simulink library "carnot"  (R2018b)
settings: Solver=VariableStepAuto  StartTime=0.0  StopTime=10.0  RelTol=1e-3
undefined symbols (not defined in the file or in its folder): A, A_earth, acol, Acol, ActPower1, ActPower2, ActPower3, Ad, Ad0, Ar, Au, Au0, Azimuth_Angle, B, Bd, Bd0, Br, Bu, Bu0, C, c1, c2, c3, c33, c4, c5, c6, CarnotCallbacks_Density, CarnotCallbacks_Enthalpy, CarnotCallbacks_Enthalpy2Temperature, CarnotCallbacks_Entropy, CarnotCallbacks_Evaporation_Enthalpy, CarnotCallbacks_GlobalMessageLevel, CarnotCallbacks_Grashof, CarnotCallbacks_Heat_Capacity, CarnotCallbacks_Kinematic_Viscosity, CarnotCallbacks_PMV_PPD, CarnotCallbacks_Prandtl, CarnotCallbacks_Saturation_Property, CarnotCallbacks_Saturation_Temperature, CarnotCallbacks_Saturation_Value_Water, CarnotCallbacks_Specific_Volume, CarnotCallbacks_Thermal_Conductivity, CarnotCallbacks_Vapour_Content, CarnotCallbacks_Vapour_Pressure, Cd, Cdl, Cr, Cu, Davies, Dd, DE_TRY2010_04_averageYear, delta_grd, density, DiameterLastPiece, dl, DPConstant, DPLinear, DPQuadratic, Dr ... (+59)
libraries: $bdroot x429, simulink x36, simulink_extras x12
(part 4 of 22)

== system carnot/Basic/Electric ==
  EBCreator : Subsystem  InitFcn=load('EB.mat');  mask(EBCreator){Inport_ID=on, Inport_f=on, Inport_v1=on, Inport_p1=on, Inport_pf1=on, Inport_v2=on, Inport_p2=on, Inport_pf2=on, Inport_v3=on, Inport_p3=on, Inport_pf3=on, ID=4, f=50, v1=230, p1=0, pf1=1, v2=230, p2=0, pf2=1, v3=230, p3=0, pf3=1, Annotation_ID=off, Annotation_f=off, Annotation_v1=off, Annotation_p1=off, Annotation_pf1=off, Annotation_v2=off, Annotation_p2=off, Annotation_pf2=off, Annotation_v3=off, Annotation_p3=off, Annotation_pf3=on}
      mask prompts: Inport_ID "ID as inport"; Inport_f "frequency as inport"; Inport_v1 "voltage line 1 as inport"; Inport_p1 "active power line 1 as inport"; Inport_pf1 "power factor line 1 as inport"; Inport_v2 "voltage line 2 as inport"; Inport_p2 "active power line 1 as inport"; Inport_pf2 "power factor line 2 as inport"; Inport_v3 "voltage line 3 as inport"; Inport_p3 "active power line 3 as inport"; Inport_pf3 "power factor line 3 as inport"; ID "ID [1]"; f "frequency [Hz]"; v1 "voltage line 1 [V]"; p1 "active power line 1 [W]"; pf1 "power factor line 1 [1]"; v2 "voltage line 2 [V]"; p2 "active power line 2 [W]"; pf2 "power factor line 2 [1]"; v3 "voltage line 3 [V]"; p3 "active power line 3 [W]"; pf3 "power factor line 3 [1]"; Annotation_ID "ID as annotation"; Annotation_f "Frequency as annotation"; Annotation_v1 "voltage line 1 as annotation"; Annotation_p1 "active power line 1 as annotation"; Annotation_pf1 "fluid type as annotation"; Annotation_v2 "voltage line 2 as annotation"; Annotation_p2 "active power line 2 as annotation"; Annotation_pf2 "power factor line 2 as annotation"; Annotation_v3 "voltage line 3 as annotation"; Annotation_p3 "voltage line 3 as annotation"; Annotation_pf3 "power factor line 3 as annotation"
      mask help:
      | This block creates an EB from input signals.
      | ID is:
      | 1  Power only
      | 2  DC
      | 3  AC_1Phase
      | 4  AC_3Phase
      mask init:
      | CarnotCallbacks_EBCreator('CreateInports', gcb);
      mask Help: web(fullfile(path_carnot('help'),'EBCreator.html'),'-helpbrowser')
      mask Callback Inport_ID:
      | CarnotCallbacks_EBCreator('CreateMaskVisibilities', gcb);
      | CarnotCallbacks_EBCreator('CreateMaskAnnotations', gcb);
      mask Callback Inport_f:
      | CarnotCallbacks_EBCreator('CreateMaskVisibilities', gcb);
      | CarnotCallbacks_EBCreator('CreateMaskAnnotations', gcb);
      mask Callback Inport_v1:
      | CarnotCallbacks_EBCreator('CreateMaskVisibilities', gcb);
      | CarnotCallbacks_EBCreator('CreateMaskAnnotations', gcb);
      mask Callback Inport_p1:
      | CarnotCallbacks_EBCreator('CreateMaskVisibilities', gcb);
      | CarnotCallbacks_EBCreator('CreateMaskAnnotations', gcb);
      mask Callback Inport_pf1:
      | CarnotCallbacks_EBCreator('CreateMaskVisibilities', gcb);
      | CarnotCallbacks_EBCreator('CreateMaskAnnotations', gcb);
      mask Callback Inport_v2:
      | CarnotCallbacks_EBCreator('CreateMaskVisibilities', gcb);
      | CarnotCallbacks_EBCreator('CreateMaskAnnotations', gcb);
      mask Callback Inport_p2:
      | CarnotCallbacks_EBCreator('CreateMaskVisibilities', gcb);
      | CarnotCallbacks_EBCreator('CreateMaskAnnotations', gcb);
      mask Callback Inport_pf2:
      | CarnotCallbacks_EBCreator('CreateMaskVisibilities', gcb);
      | CarnotCallbacks_EBCreator('CreateMaskAnnotations', gcb);
      mask Callback Inport_v3:
      | CarnotCallbacks_EBCreator('CreateMaskVisibilities', gcb);
      | CarnotCallbacks_EBCreator('CreateMaskAnnotations', gcb);
      mask Callback Inport_p3:
      | CarnotCallbacks_EBCreator('CreateMaskVisibilities', gcb);
      | CarnotCallbacks_EBCreator('CreateMaskAnnotations', gcb);
      mask Callback Inport_pf3:
      | CarnotCallbacks_EBCreator('CreateMaskVisibilities', gcb);
      | CarnotCallbacks_EBCreator('CreateMaskAnnotations', gcb);
      mask Callback ID: CarnotCallbacks_EBCreator('CreateMaskAnnotations', gcb);
      mask Callback f: CarnotCallbacks_EBCreator('CreateMaskAnnotations', gcb);
      mask Callback v1: CarnotCallbacks_EBCreator('CreateMaskAnnotations', gcb);
      mask Callback p1: CarnotCallbacks_EBCreator('CreateMaskAnnotations', gcb);
      mask Callback pf1: CarnotCallbacks_EBCreator('CreateMaskAnnotations', gcb);
      mask Callback v2: CarnotCallbacks_EBCreator('CreateMaskAnnotations', gcb);
      mask Callback p2: CarnotCallbacks_EBCreator('CreateMaskAnnotations', gcb);
      mask Callback pf2: CarnotCallbacks_EBCreator('CreateMaskAnnotations', gcb);
      mask Callback v3: CarnotCallbacks_EBCreator('CreateMaskAnnotations', gcb);
      mask Callback p3: CarnotCallbacks_EBCreator('CreateMaskAnnotations', gcb);
      mask Callback pf3: CarnotCallbacks_EBCreator('CreateMaskAnnotations', gcb);
      mask Callback Annotation_ID: CarnotCallbacks_EBCreator('CreateMaskAnnotations', gcb);
      mask Callback Annotation_f: CarnotCallbacks_EBCreator('CreateMaskAnnotations', gcb);
      mask Callback Annotation_v1: CarnotCallbacks_EBCreator('CreateMaskAnnotations', gcb);
      mask Callback Annotation_p1: CarnotCallbacks_EBCreator('CreateMaskAnnotations', gcb);
      mask Callback Annotation_pf1: CarnotCallbacks_EBCreator('CreateMaskAnnotations', gcb);
      mask Callback Annotation_v2: CarnotCallbacks_EBCreator('CreateMaskAnnotations', gcb);
      mask Callback Annotation_p2: CarnotCallbacks_EBCreator('CreateMaskAnnotations', gcb);
      mask Callback Annotation_pf2: CarnotCallbacks_EBCreator('CreateMaskAnnotations', gcb);
      mask Callback Annotation_v3: CarnotCallbacks_EBCreator('CreateMaskAnnotations', gcb);
      mask Callback Annotation_p3: CarnotCallbacks_EBCreator('CreateMaskAnnotations', gcb);
      mask Callback Annotation_pf3: CarnotCallbacks_EBCreator('CreateMaskAnnotations', gcb);
      mask DialogControl ParameterTabVar0 Prompt: Settings
      mask DialogControl ParameterTabVar01 Prompt: Values
      mask DialogControl ParameterTabVar012 Prompt: Annotations
  basic_EB : Subsystem  InitFcn=load('EB.mat')  mask(basic_EB){eID=Power only, f=50, v1=230, p1=0, pf1=1, v2=230, p2=0, pf2=1, v3=230, p3=0, pf3=1}
      mask prompts: eID "ID for electric calculation"; f "frequency [Hz]"; v1 "voltage to ground [V]"; p1 "active  power [VA]"; pf1 "power factor[-]"; v2 "voltage to ground [V]"; p2 "active  power [VA]"; pf2 "power factor[-]"; v3 "voltage to ground [V]"; p3 "active  power [VA]"; pf3 "power factor[-]"
      mask help: Create a constant Electric Bus.
      mask Help: web(fullfile(path_carnot('help'),'basic_EB.html'),'-helpbrowser')
      mask TypeOptions eID: ID/eID
      mask TypeOptions f: f/Value
      mask TypeOptions v1: v1/Value
      mask TypeOptions p1: p1/Value
      mask TypeOptions pf1: pf1/Value
      mask TypeOptions v2: v2/Value
      mask TypeOptions p2: p2/Value
      mask TypeOptions pf2: pf2/Value
      mask TypeOptions v3: v3/Value
      mask TypeOptions p3: p3/Value
      mask TypeOptions pf3: pf3/Value
      mask DialogControl ParameterTabVar03 Prompt: Common
      mask DialogControl ParameterTabVar0 Prompt: Line 1
      mask DialogControl ParameterTabVar01 Prompt: Line2
      mask DialogControl ParameterTabVar02 Prompt: Line3
  basic_create_EB : Subsystem  InitFcn=load('EB.mat')  mask(basic_create_EB){eID=Power only, f=50, pf1=1, pf2=1, pf3=1}
      mask prompts: eID "ID for electric calculation"; f "frequency [Hz]"; pf1 "power factor line 1 [-]"; pf2 "power factor line 2 [-]"; pf3 "power factor line 3 [-]"
      mask help: Block to create an EB with the variable inputs ActPower and Voltage. The other values can be set as constants in the mask.
      mask Help: web(fullfile(path_carnot('help'),'basic_create_EB.html'),'-helpbrowser')
      mask TypeOptions eID: basic_EB/eID
      mask TypeOptions f: basic_EB/f
      mask TypeOptions pf1: basic_EB/pf1
      mask TypeOptions pf2: basic_EB/pf2
      mask TypeOptions pf3: basic_EB/pf3

== system carnot/Basic/Heat_Transfer ==
  HeatTransfer2Ground_ISO13370 : Subsystem  mask(Heat Transfer to Ground ISO 13370){slabwidth=10, slablength=7, gammat=0, Tmeaninside=23.8, deltathetai=3.8, Tmeanoutside=11, deltathetae=9.3, tshift=319*3600, dwall=0.4, cond_ground=2.0, cp_ground=800, rho_ground=2500, utot=0.183}
      mask prompts: slabwidth "Width of slab in m"; slablength "Length of slab in m"; gammat "Linear thermal transmittance associated with wall/floor junctions [W/mK]"; Tmeaninside "Mean annual inside temperature [°C]"; deltathetai "Annual amplitude of inside temperature [°C]"; Tmeanoutside "Mean annual outside temperature [°C]"; deltathetae "Annual amplitude of outside temperature [°C]"; tshift "Time shift where outside temperature sine-curve shows a mimimum [s]"; dwall "Average thickness of walls inlcuding all layers [m]"; cond_ground "Conductivity of ground [W/(m*K)]"; cp_ground "Capacity of ground [J/(kg*K)]"; rho_ground "Density of ground [kg/m^3]"; utot "Total heat transfer of slab to ground [W/m²/K]"
      mask help:
      | Ground heat transfer for a floor "SLAB ON GROUND" according to ISO 13370:2007.
      | Use function fitSineToTamb to find the weather parameters.
      mask Help: web(fullfile(path_carnot('help'),'Heattransfer2GroundISO.html'),'-helpbrowser')
      mask Display: disp('U(ground)\nISO13370')
  HeatTransfer2Ground_Simple : Subsystem  mask(Heat Transfer to Ground simple Model){Tground=10, UAground=0.2*70}
      mask prompts: Tground "Ground temperature in °C"; UAground "Heat transfer to ground in W/K"
      mask help:
      | Very simple model for the heat transfer of a house to the ground.
      | See Help for details.
      mask Help: web(fullfile(path_carnot('help'),'Heattransfer2Ground_Simple.html'),'-helpbrowser')
  alfa_ceiling : Subsystem  mask(ALFA){active=0, emission_c=0.65, wallsurface=1}
      mask prompts: active "active layer (0 / 1)"; emission_c "Longwave emissivity of surface (0..1)"; wallsurface "Ceiling surface in m²"
      mask help:
      | Convective and radiative heat transfer at the SURFACE OF A HORIZONTAL CEELING.
      | [AIV] : conditions of zone node,
      | Ts : temperature of outdoor wall surface, °C,
      | qdots : specific heat flow into wall construction, W/m^2,
      | [S] : heat and air flow to zone node.
      mask Help: web(fullfile(path_carnot('help'),'alfa_ceiling.html'),'-helpbrowser')
  alfa_floor : Subsystem  mask(ALFA){active=0, emission_f=0.65, wallsurface=1}
      mask prompts: active "active layer (0 / 1)"; emission_f "Longwave emissivity of surface (0..1)"; wallsurface "Floor surface in m²"
      mask help:
      | Convective and radiative heat transfer at the SURFACE OF A HORIZONTAL FLOOR.
      |
      | [AIV] : conditions of zone node,
      | Ts : temperature of wall surface, °C,
      | qdots : specific heat flow into wall construction, W/m^2,
      | [S] : heat and air flow to zone node.
      mask Help: web(fullfile(path_carnot('help'),'alfa_floor.html'),'-helpbrowser')
  alfa_wall_in : Subsystem  mask(ALFA){active=0, emission_in=0.7, wallsurface=1}
      mask prompts: active "Active layer (0 / 1)"; emission_in "Longwave emissivity of surface (0..1)"; wallsurface "Wall surface in m²"
      mask help:
      | Convective and radiative heat transfer at the INDOOR SURFACE of a VERTICAL OUTER WALL.
      |
      | [AIV] : conditions of zone node,
      | Ts : temperature of wall surface, °C,
      | qdots : specific heat flow into wall construction, W/m^2,
      | [S] : heat and air flow to zone node.
      mask Help: web(fullfile(path_carnot('help'),'alfa_wall_in.html'),'-helpbrowser')
  alfa_wall_out : Subsystem  mask(ALFA){pos=0, absorption_out=0.4, emission_out=0.7, wallsurface=1}
      mask prompts: pos "Azimut (south = 0, east = -90) in degrees"; absorption_out "Solar absorption outside (0..1)"; emission_out "Longwave emissivity of surface (0..1)"; wallsurface "Wall surface in m²"
      mask help:
      | Convective and radiative HEAT TRANSFER at the WEATHER EXPOSED SURFACE of an OUTER WALL.
      |
      | [W*] : modified weather data, adapted to height over ground,
      | Ts : temperature of outdoor wall surface, °C,
      | qdots : specific heat flow into wall / window construction, W/m^2.
      mask init:
      | if length(pos) == 1
      |     pos = [90  pos 0]; % pos is [inclination azimut rotation]
      | end
      mask Help: web(fullfile(path_carnot('help'),'alfa_wall_out.html'),'-helpbrowser')
  alfa_window_in : Subsystem  mask(ALFA){type_glazing=double glazing normal, gvalue=0.7, tauzero=0.8, emission_in=1, wallsurface=1, frame=0.1, numlayer=2, shad_type=No shading, tau_shad=0.01, bli_a=0.05, bli_b=1, bli_c=0.05, bli_d=0.05, bli_alpha=90, bli_refl=0.2}
      mask prompts: type_glazing "glazing type"; gvalue "Energy transmission by sunlight (g-value) 0..1"; tauzero "transmittance in visible range of the sunlight [0..1]"; emission_in "Longwave emissivity (0..1)"; wallsurface "Surface of the window (with frame) in m²"; frame "Share of the frame on the surface (0...1)"; numlayer "Number of glass panes"; shad_type "shading type [no Shading/exterior/interior]"; tau_shad "solar transmittance of shading element [0..1]"; bli_a "a  Depth of blind blades [m]"; bli_b "b heigth of blind blades [m]"; bli_c "c distance of "b" to back end of blind blade [m]"; bli_d "d offset between blind blades [m]"; bli_refl "optical reflectance of blind surface [0..1]"
      mask help:
      | Convective and radiative heat transfer at the INDOOR SURFACE OF A VERTICAL WINDOW with 1-4 layers (each 3 ... 8 mm thick).
      |
      | Ts  : temperature of window surface, °C,
      | [sun_t]  : sun data (incidence angle, direct and diffuse radiation
      |     at tilted window surface),
      | [AIV]  : conditions of zone node,
      | qdots  : specific heat flow into window construction, W/m^2,
      | qdot_abs : specific irradiation absorption within window
      |     construction,  W/m^2,
      | [S]  : heat and air flow to zone node.
      mask Help: web(fullfile(path_carnot('help'),'alfa_window_in.html'),'-helpbrowser')
      mask TypeOptions type_glazing: double glazing normal | double glazing  thermal insulation | double glazing combi 73/41 | double glazing combi 50/24 | triple glazing normal | triple glazing  thermal insulation
      mask TypeOptions tauzero: Subsystem/tau(0)/Gain
      mask TypeOptions shad_type: No shading | Exterior Screen | Interior Screen | Venetian Blind
  alfa_window_out : Subsystem  mask(ALFA){pos=0, absorption_out=0.01, emission_out=0.87, frame=0.1}
      mask prompts: pos "Azimut of the surface (South = 0; East = -90)"; absorption_out "Solar absorption of the glass (0...1)"; emission_out "Longwave emissivity (0...1)"; frame "Share of the frame on the surface (0..1)"
      mask help:
      | Convective and radiative heat transfer at the OUTDOOR SURFACE OF A VERTICAL WINDOW.
      | Azimut can be a scalar or a vector with [inclination azimut rotation].
      | [WDB] weather data bus, adapted to height over ground,
      | Ts : temperature of outdoor window surface, °C,
      | g : energetic solar radiation transmittance
      | qdots : specific heat flow into window construction, W/m^2,
      | [sun_t] : sun data (incidence angle, direct and diffuse radiation at tilted window surface).
      mask init:
      | if length(pos) == 1
      |     pos = [90  pos 0]; % pos is [inclination azimut rotation]
      | end
      mask Help: web(fullfile(path_carnot('help'),'alfa_window_out.html'),'-helpbrowser')
  wall_out_IR_radiation : Subsystem

== system carnot/Basic/Hydraulics ==
  ElectricConsumptionPump : Subsystem  mask(Electric Consumption of a Pump){e0=10, e1=10, e2=-1}
      mask prompts: e0 "e0: constant coefficient in W"; e1 "e1: linear coefficient in W*s/kg"; e2 "e2: quadratic coefficient in W*(s/kg)²"
      mask help:
      | The electric consumption of the pump is given by the quadratic equation
      |   Pel = e0 + e1*mdot + e2*mdot^2
      | with
      |   mdot : massflow in kg/s
      |   Pel : electric consumption in W
      mask TypeOptions e0: Constant/Value
      mask TypeOptions e1: Linear/Gain
      mask TypeOptions e2: Quadratic/Gain
      mask Display: disp('Pel = e0\n+ e1*mdot\n+ e2*mdot² ')
  Flow_Mixer_basic : Subsystem  mask(Flow Mixer Basic){}
      mask help:
      | The flow mixer calculated the temperature and massflow of 2 entering flows.
      | The temperature is calculated in the block Mix_T_Mdot.
      | The flow diversion fdiv (feed back to the flow diverter) takes care that the pressure drop in the 2 branches is the same. The resulting pressure drop coefficients are calulated in the s-function mix_flow (uses solve_quadratic_equation in Carlib).
      mask Help: web(fullfile(path_carnot('help'),'Flow_Mixer_basic.html'),'-helpbrowser')
      mask Display: disp('Flow\nMixer')
  Grashof : Subsystem  LoadFcn=CarnotCallbacks_Grashof('LoadFcn');  VariantControl=CarlibClassic  mask(Grashof){DEBUGLEVEL=WARNINGLEVEL, MAXTOTALMESSAGES=inf, MAXCONSECUTIVEMESSAGES=inf, WRITETOFILE=0, FILENAME='errors.txt'}
      mask prompts: DEBUGLEVEL "Debug level"; MAXTOTALMESSAGES "maximum number of total warning"; MAXCONSECUTIVEMESSAGES "maximum number of consecutive warnings"; WRITETOFILE "write messages to file"; FILENAME "filename for error messages"
      mask help:
      | Calculates the Gashof number. You may use the block "GlobalMessageLevel" in the Toolbox to handle the debugging messages.
      | Inputs are:
      | 1   wall temperature - scalar or vector
      | 2   temperature at infinite distance - scalar
      | 3   pressure - scalar
      | 4   fluid type (see below) - scalar
      | 5   fluid_mix - scalar
      | 6   characteristic dimension - scalar
      |
      | FluidType        Remarks
      | 1: water          fluid mix is vapourcontent in the 2-phase region
      | 2: air              fluid mix is (kg water) / (kg dry air)
      | 3: cotton oil       -
      | 4: silicone oil     -
      | 5: water-glycol   fluid mix is volume partition [0..1] of propylen glycol
      | 6: Tyfocor LS     function only available in liquid phase
      | 7: Water Constant = water at 20°C
      | 8: Air Constant = air at 20°C
      mask init:
      | %global debug level
      | [DEBUGLEVEL, MAXTOTALMESSAGES, MAXCONSECUTIVEMESSAGES, WRITETOFILE, FILENAME] = CarnotCallbacks_Grashof('CheckDebugLevels', DEBUGLEVEL, MAXTOTALMESSAGES, MAXCONSECUTIVEMESSAGES, WRITETOFILE, FILENAME);
      mask Help: web(fullfile(path_carnot('help'),'Grashof_mdl.html'),'-helpbrowser')
      mask TypeOptions DEBUGLEVEL: DEBUGLEVEL | INFOLEVEL | WARNINGLEVEL | ERRORLEVEL | FATALLEVEL | NOLEVEL
      mask DialogControl ParameterTabVar0 Prompt: Debugging
  Mix_T_Mdot : Subsystem  InitFcn=load('THB.mat');  mask(mix_temperature){mixcalc=Tmix = (mdot1*T1 + mdot2*T2)/(mdot1+mdot2)}
      mask prompts: mixcalc "Calculation of mixture :"
      mask help:
      | Calculate the temperature of the mixture of two flows. Uses enthalpy balance for humid air. Liquids may be mixed by the (faster and approximate) equation:
      | Tmix = (mdot1*T1 + mdot2*T2)/(mdot1+mdot2)
      mask Help: web(fullfile(path_carnot('help'),'Mix_T_Mdot.html'),'-helpbrowser')
      mask TypeOptions mixcalc: Tmix = (mdot1*T1 + mdot2*T2)/(mdot1+mdot2) | Enthalpy balance
  Prandtl : Subsystem  LoadFcn=CarnotCallbacks_Prandtl('LoadFcn');  InitFcn=load('THB.mat');  VariantControl=CarlibClassic  mask(Prandtl){INPUTARGUMENTS=state variables (classic), DEBUGLEVEL=WARNINGLEVEL, MAXTOTALMESSAGES=inf, MAXCONSECUTIVEMESSAGES=inf, WRITETOFILE=0, FILENAME='errors.txt'}
      mask prompts: INPUTARGUMENTS "Input arguments"; DEBUGLEVEL "Debug level"; MAXTOTALMESSAGES "maximum number of total warning"; MAXCONSECUTIVEMESSAGES "maximum number of consecutive warnings"; WRITETOFILE "write messages to file"; FILENAME "filename for error messages"
      mask help:
      | Calculates the Prandtl number for given materials properties.
      | You may use the block "GlobalMessageLevel" in the Toolbox to handle the debugging messages.
      | FluidType        Remarks
      | 1: water          fluid mix is vapourcontent in the 2-phase region
      | 2: air              fluid mix is (kg water) / (kg dry air)
      | 3: cotton oil       -
      | 4: silicone oil     -
      | 5: water-glycol   fluid mix is volume partition [0..1] of propylen glycol
      | 6: Tyfocor LS     function only available in liquid phase
      | 7: Water Constant = 998.21 kg/m³ (water at 20°C)
      | 8: Air Constant   = 1.118 kg/m³ (air at 20°C)
      mask init:
      | %Inports
      | CarnotCallbacks_Prandtl('CreateInports');
      | 
      | %global debug level
      | [DEBUGLEVEL, MAXTOTALMESSAGES, MAXCONSECUTIVEMESSAGES, WRITETOFILE, FILENAME] = CarnotCallbacks_Prandtl('CheckDebugLevels', DEBUGLEVEL, MAXTOTALMESSAGES, MAXCONSECUTIVEMESSAGES, WRITETOFILE, FILENAME);
      mask Help: web(fullfile(path_carnot('help'),'Prandtl_mdl.html'),'-helpbrowser')
      mask TypeOptions INPUTARGUMENTS: state variables (classic) | THB | THV
      mask Callback INPUTARGUMENTS: CarnotCallbacks_Prandtl('MaskVisibilities');
      mask TypeOptions DEBUGLEVEL: DEBUGLEVEL | INFOLEVEL | WARNINGLEVEL | ERRORLEVEL | FATALLEVEL | NOLEVEL
      mask DialogControl ParameterTabVar0 Prompt: Parameters
      mask DialogControl ParameterTabVar01 Prompt: Debugging
  Reynolds : Subsystem  mask(Reynolds number){}
      mask help:
      | Calculates the Reynolds number for a flow, give the characteristic dimension as an input.
      | Pipe: diameter
      | Duct: 4 * cross_section / perimeter
      | Plate: length
      mask Help: web(fullfile(path_carnot('help'),'Reynolds_mdl.html'),'-helpbrowser')
  ReynoldsTHB : Subsystem  mask(Reynolds THB){}
      mask help: Calculates the Reynolds number for pipes with round cross-section.
      mask Help: web(fullfile(path_carnot('help'),'ReynoldsTHB.html'),'-helpbrowser')
  THBCreator : Subsystem  InitFcn=load('THB.mat');  mask(THBCreator){Inport_ID=on, Inport_T=on, Inport_mdot=on, Inport_p=on, Inport_type=on, Inport_mix=on, Inport_mix2=on, Inport_mix3=on, Inport_d=on, Inport_c=on, Inport_l=on, Inport_q=on, Inport_LH=on, Inport_H=on, ID=20001, T=20, mdot=0, p=1e5, FluidType=1, FluidMix=0, FluidMix2=0, FluidMix3=0, d=0.02, c=0, l=0, q=0, LH=0, H=0, Annotation_ID=off, Annotation_T=off, Annotation_mdot=off, Annotation_p=off, Annotation_type=off, Annotation_mix=off, Annotation_mix2=off, Annotation_mix3=off, Annotation_d=off, Annotation_c=off, Annotation_l=off, Annotation_q=off, Annotation_LH=off, Annotation_H=off}
      mask prompts: Inport_ID "ID as inport"; Inport_T "temperature as inport"; Inport_mdot "mass flow rate as inport"; Inport_p "pressure as inport"; Inport_type "fluid type as inport"; Inport_mix "fluid mix as inport"; Inport_mix2 "fluid mix2 as inport"; Inport_mix3 "fluid mix3 as inport"; Inport_d "diameter last piece as inport"; Inport_c "constant pressure drop coefficient as inport"; Inport_l "linear pressure drop coefficient as inport"; Inport_q "quadratic pressure drop coefficient as inport"; Inport_LH "hydraulic inductance as inport"; Inport_H "geodetic height as inport"; ID "ID [1]"; T "temperature [°C]"; mdot "mass flow rate [kg/s]"; p "pressure [Pa]"; FluidType "fluid type [enum]"; FluidMix "fluid mix [1]"; FluidMix2 "fluid mix [2]"; FluidMix3 "fluid mix [3]"; d "diameter last piece [m]"; c "constant pressure drop coefficient [Pa]"; l "linear pressure drop coefficient [Pa/(kg/s)]"; q "quadratic pressure drop coefficient [Pa/(kg/s)²]"; LH "hydraulic inductance [1/m]"; H "geodetic height"; Annotation_ID "ID as annotation"; Annotation_T "temperature as annotation"; Annotation_mdot "mass flow rate as annotation"; Annotation_p "pressure as annotation"; Annotation_type "fluid type as annotation"; Annotation_mix "fluid mix as annotation"; Annotation_mix2 "fluid mix2 as annotation"; Annotation_mix3 "fluid mix3 as annotation"; Annotation_d "diameter last piece as annotation"; Annotation_c "constant pressure drop coefficient as annotation"; Annotation_l "linear pressure drop coefficient as annotation"; Annotation_q "quadratic pressure drop coefficient as annotation"; Annotation_LH "hydraulic inductance as annotation"; Annotation_H "geodetic height as annotation"
      mask help: This block creates a THB from input signals.
      mask init:
      | CarnotCallbacks_THBCreator('CreateInports', gcb);
      mask Help: web(fullfile(path_carnot('help'),'THBCreator.html'),'-helpbrowser')
      mask Callback Inport_ID:
      | CarnotCallbacks_THBCreator('CreateMaskVisibilities', gcb);
      | CarnotCallbacks_THBCreator('CreateMaskAnnotations', gcb);
      mask Callback Inport_T:
      | CarnotCallbacks_THBCreator('CreateMaskVisibilities', gcb);
      | CarnotCallbacks_THBCreator('CreateMaskAnnotations', gcb);
      mask Callback Inport_mdot:
      | CarnotCallbacks_THBCreator('CreateMaskVisibilities', gcb);
      | CarnotCallbacks_THBCreator('CreateMaskAnnotations', gcb);
      mask Callback Inport_p:
      | CarnotCallbacks_THBCreator('CreateMaskVisibilities', gcb);
      | CarnotCallbacks_THBCreator('CreateMaskAnnotations', gcb);
      mask Callback Inport_type:
      | CarnotCallbacks_THBCreator('CreateMaskVisibilities', gcb);
      | CarnotCallbacks_THBCreator('CreateMaskAnnotations', gcb);
      mask Callback Inport_mix:
      | CarnotCallbacks_THBCreator('CreateMaskVisibilities', gcb);
      | CarnotCallbacks_THBCreator('CreateMaskAnnotations', gcb);
      mask Callback Inport_mix2:
      | CarnotCallbacks_THBCreator('CreateMaskVisibilities', gcb);
      | CarnotCallbacks_THBCreator('CreateMaskAnnotations', gcb);
      mask Callback Inport_mix3:
      | CarnotCallbacks_THBCreator('CreateMaskVisibilities', gcb);
      | CarnotCallbacks_THBCreator('CreateMaskAnnotations', gcb);
      mask Callback Inport_d:
      | CarnotCallbacks_THBCreator('CreateMaskVisibilities', gcb);
      | CarnotCallbacks_THBCreator('CreateMaskAnnotations', gcb);
      mask Callback Inport_c:
      | CarnotCallbacks_THBCreator('CreateMaskVisibilities', gcb);
      | CarnotCallbacks_THBCreator('CreateMaskAnnotations', gcb);
      mask Callback Inport_l:
      | CarnotCallbacks_THBCreator('CreateMaskVisibilities', gcb);
      | CarnotCallbacks_THBCreator('CreateMaskAnnotations', gcb);
      mask Callback Inport_q:
      | CarnotCallbacks_THBCreator('CreateMaskVisibilities', gcb);
      | CarnotCallbacks_THBCreator('CreateMaskAnnotations', gcb);
      mask Callback Inport_LH:
      | CarnotCallbacks_THBCreator('CreateMaskVisibilities', gcb);
      | CarnotCallbacks_THBCreator('CreateMaskAnnotations', gcb);
      mask Callback Inport_H:
      | CarnotCallbacks_THBCreator('CreateMaskVisibilities', gcb);
      | CarnotCallbacks_THBCreator('CreateMaskAnnotations', gcb);
      mask Callback ID: CarnotCallbacks_THBCreator('CreateMaskAnnotations', gcb);
      mask Callback T: CarnotCallbacks_THBCreator('CreateMaskAnnotations', gcb);
      mask Callback mdot: CarnotCallbacks_THBCreator('CreateMaskAnnotations', gcb);
      mask Callback p: CarnotCallbacks_THBCreator('CreateMaskAnnotations', gcb);
      mask Callback FluidType: CarnotCallbacks_THBCreator('CreateMaskAnnotations', gcb);
      mask Callback FluidMix: CarnotCallbacks_THBCreator('CreateMaskAnnotations', gcb);
      mask Callback FluidMix2: CarnotCallbacks_THBCreator('CreateMaskAnnotations', gcb);
      mask Callback FluidMix3: CarnotCallbacks_THBCreator('CreateMaskAnnotations', gcb);
      mask Callback d: CarnotCallbacks_THBCreator('CreateMaskAnnotations', gcb);
      mask Callback c: CarnotCallbacks_THBCreator('CreateMaskAnnotations', gcb);
      mask Callback l: CarnotCallbacks_THBCreator('CreateMaskAnnotations', gcb);
      mask Callback q: CarnotCallbacks_THBCreator('CreateMaskAnnotations', gcb);
      mask Callback LH: CarnotCallbacks_THBCreator('CreateMaskAnnotations', gcb);
      mask Callback H: CarnotCallbacks_THBCreator('CreateMaskAnnotations', gcb);
      mask Callback Annotation_ID: CarnotCallbacks_THBCreator('CreateMaskAnnotations', gcb);
      mask Callback Annotation_T: CarnotCallbacks_THBCreator('CreateMaskAnnotations', gcb);
      mask Callback Annotation_mdot: CarnotCallbacks_THBCreator('CreateMaskAnnotations', gcb);
      mask Callback Annotation_p: CarnotCallbacks_THBCreator('CreateMaskAnnotations', gcb);
      mask Callback Annotation_type: CarnotCallbacks_THBCreator('CreateMaskAnnotations', gcb);
      mask Callback Annotation_mix: CarnotCallbacks_THBCreator('CreateMaskAnnotations', gcb);
      mask Callback Annotation_mix2: CarnotCallbacks_THBCreator('CreateMaskAnnotations', gcb);
      mask Callback Annotation_mix3: CarnotCallbacks_THBCreator('CreateMaskAnnotations', gcb);
      mask Callback Annotation_d: CarnotCallbacks_THBCreator('CreateMaskAnnotations', gcb);
      mask Callback Annotation_c: CarnotCallbacks_THBCreator('CreateMaskAnnotations', gcb);
      mask Callback Annotation_l: CarnotCallbacks_THBCreator('CreateMaskAnnotations', gcb);
      mask Callback Annotation_q: CarnotCallbacks_THBCreator('CreateMaskAnnotations', gcb);
      mask Callback Annotation_LH: CarnotCallbacks_THBCreator('CreateMaskAnnotations', gcb);
      mask Callback Annotation_H: CarnotCallbacks_THBCreator('CreateMaskAnnotations', gcb);
      mask DialogControl ParameterTabVar0 Prompt: Settings
      mask DialogControl ParameterTabVar01 Prompt: Values
      mask DialogControl ParameterTabVar012 Prompt: Annotations
  Velocity : Subsystem  mask(velocity){}
      mask help: Calculates the velocity in a pipe [m/s] assuming a round pipe. The diameter is taken from the THV-vector.
      mask Help: web(fullfile(path_carnot('help'),'Velocity_mdl.html'),'-helpbrowser')
  basic_THB : Subsystem  InitFcn=load('THB.mat');  mask(basic THB){t=20, mdot=0, p=1e5, ID=Pressure Drop from Massflow, fluid=Water, mix=0, mix2=0, mix3=0, dia=0.02, hgt=0}
      mask prompts: t "temperature [°C]"; mdot "massflow [kg/s]"; p "pressure [Pa]"; ID "ID for pressure drop calculation"; mix "fluid mixture [0..1]"; mix2 "fluid mixture 2 [0..1]"; mix3 "fluid mixture 3 [0..1]"; dia "diameter [m]"; hgt "Static height in m"
      mask help:
      | Create a constant Thermo-Hydraulic-Vector.
      | Pressure drop calculation mode (defined by ID):
      |     1 ..  9999 no pressure drop (dp)
      | 10001 .. 19999 dp caused by flowrate
      | 20001 .. inf   dp by flowrate and static height
      mask Help: web(fullfile(path_carnot('help'),'basic_THB.html'),'-helpbrowser')
      mask TypeOptions t: const24/Value
      mask TypeOptions mdot: const25/Value
      mask TypeOptions p: const26/Value
      mask TypeOptions ID: const21/mID
      mask TypeOptions fluid: const27/fluid
      mask TypeOptions mix: const28/Value
      mask TypeOptions mix2: const2/Value
      mask TypeOptions mix3: const3/Value
      mask TypeOptions dia: const29/Value
      mask TypeOptions hgt: const1/Value
      mask DialogControl ParameterTabVar0 Prompt: Hydraulic
      mask DialogControl ParameterTabVar01 Prompt: Fluid
      mask DialogControl ParameterTabVar012 Prompt: Geometry
  basic_create_THB : Subsystem  InitFcn=load('THB.mat');  mask(basic create THB){p=2e5, fluid=Water, mix=0, mix2=0, mix3=0, dia=0.03, hgt=0, mID=No Pressure Drop}
      mask prompts: p "pressure [Pa]"; mix "fluid mixture [0..1]"; mix2 "fluid mixture 2 [0..1]"; mix3 "fluid mixture 3 [0..1]"; dia "diameter [m]"; hgt "Static height in m"; mID "ID for pressure drop calculation"
      mask help:
      | Create a THB with the variable input T and mdot. The other value can be set as constants in the mask.
      | Pressure drop calculation mode (defined by ID):
      |     1 ..  9999 no pressure drop (dp)
      | 10001 .. 19999 dp caused by flowrate
      | 20001 .. inf   dp by flowrate and static height
      mask Help: web(fullfile(path_carnot('help'),'basic_create_THB.html'),'-helpbrowser')
      mask TypeOptions p: basic_THB/p
      mask TypeOptions fluid: basic_THB/fluid
      mask TypeOptions mix: basic_THB/mix
      mask TypeOptions mix2: basic_THB/mix2
      mask TypeOptions mix3: basic_THB/mix3
      mask TypeOptions dia: basic_THB/dia
      mask TypeOptions hgt: basic_THB/hgt
      mask TypeOptions mID: basic_THB/ID
